simulink model "Path_3D"  (R2024b)
settings: Solver=ode1  StartTime=0.0  StopTime=10.0  FixedStep=0.5e-3  RelTol=1e-3
model workspace (MAT data in the model file):
  cfg_M.ax0 = -8.7
  cfg_M.ay0 = -190.9
  cfg_M.az0 = -190.4
  cfg_M.ax1 = -23.6
  cfg_M.ay1 = -45.5
  cfg_M.az1 = -12.9
  cfg_M.ax2 = -6.9
  cfg_M.ay2 = 75.9
  cfg_M.az2 = 6826.5
  cfg_M.ax3 = -17.809705
  cfg_M.ay3 = 13.971374
  cfg_M.az3 = 1.783211
  cfg_M.bx1 = 777.2
  cfg_M.by1 = 58.9
  cfg_M.bz1 = 276.6
  cfg_M.VR = 30
  cfg_M.VT = 44.5
  cfg_M.VO = 122.870185
  cfg_M.a = 0.29
  cfg_M.b = 62.89
  cfg_M.c = 0.7
  cfg_M.d = 10.99
  cfg_M.e = 0.04
  cfg_N.BCL = 0.814
  cfg_N.SD = 0.002
  cfg_N.f1 = 0.1
  cfg_N.f2 = 0.25
  cfg_N.sigma1sq = 0.0035
  cfg_N.sigma2sq = 0.007
  cfg_N.d2 = 1281
  cfg_N.ERP = 0.1615
  cfg_N.d0 = -773.2
  cfg_N.MDP = -85.3
  cfg_N.VT = 23.81
  cfg_N.VR = 47.94
  cfg_N.Vh = -4
  cfg_N.hr = 0.1
  cfg_N.hs = 35
  cfg_N.s = 5
  cfg_N.j = 0
  cfg_N.m = 1
  cfg_N.h = 0.2
  cfg_N.f = 0.1
  cfg_N.r = 0.5
  cfg_P.CVi2j = 57
  cfg_P.Dij = 1
  cfg_P.aij = 0.01
  cfg_P.bij = 3.5
  cfg_P.cij = 0
  cfg_P.CVj2i = 57
  cfg_P.Dji = 1
  cfg_P.aji = 0.3
  cfg_P.bji = 62.89
  cfg_P.cji = 10.99
  l = 1
settings Model: DataDictionary=pathExample.sldd  Creator=wai484  LastModifiedBy=wai484
settings SolverCC: EnableFixedStepZeroCrossing=on
settings OptimizationCC: UseDivisionForNetSlopeComputation=UseDivisionForReciprocalsOfIntegersOnly

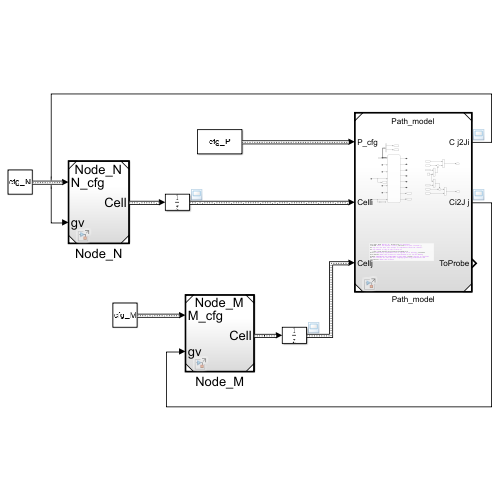
[thumbnail: Simulink's stored preview of the top-level diagram]
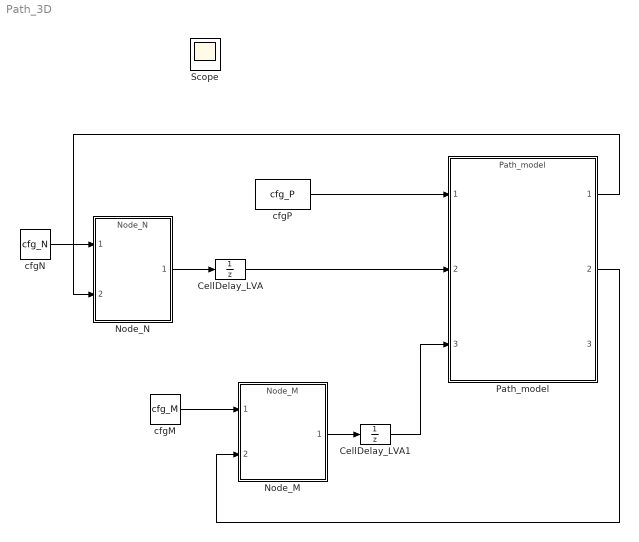
== system Path_3D ==
  CellDelay_LVA : UnitDelay  SampleTime=-1  HasFrameUpgradeWarning=on
  CellDelay_LVA1 : UnitDelay  SampleTime=-1  HasFrameUpgradeWarning=on
  Node_M : ModelReference  ModelNameDialog=Node_M  SimulationMode=Normal  ModelReferenceVersion=1.87
  Node_N : ModelReference  ModelNameDialog=Node_N  SimulationMode=Normal  ModelReferenceVersion=1.106
  Path_model : ModelReference  ModelNameDialog=Path_model.slx  ParameterArgumentNames=l  UsingDefaultArgumentValue=0  SimulationMode=Normal  ModelReferenceVersion=1.87
  cfgM : Constant  Value=cfg_M  OutDataTypeStr=Bus: Config_M
  cfgN : Constant  Value=cfg_N  OutDataTypeStr=Bus: Config_N
  cfgP : Constant  Value=cfg_P  OutDataTypeStr=Bus: Config_Path  SampleTime=-1
  Scope : Scope
  wires:
  cfgP/1 -> Path_model/1
  Node_M/1 -> CellDelay_LVA1/1
  CellDelay_LVA1/1 -> Path_model/3
  Node_N/1 -> CellDelay_LVA/1
  CellDelay_LVA/1 -> Path_model/2
  cfgN/1 -> Node_N/1
  cfgM/1 -> Node_M/1
  Path_model/2 -> Node_M/2
  Path_model/1 -> Node_N/2
